simulink model "dve_nadrze_linearized"  (R2016a)
settings: Solver=VariableStepAuto  SolverMode=SingleTasking  StartTime=0.0  StopTime=t  RelTol=1e-3
undefined symbols (not defined in the file): A, B, C, D, dQ, H1r, H2r, stepTime, U
settings Model: Creator=Filip Jašek  LastModifiedBy=Filip Jašek
settings DataIOCC: ReturnWorkspaceOutputs=on
settings DebuggingCC: SFUnexpectedBacktrackingDiag=error  SFNoUnconditionalDefaultTransitionDiag=error
settings SFSimCC: SimUseLocalCustomCode=on
settings RTWCC: RTWUseLocalCustomCode=on
settings GRTTargetCC: TargetLangStandard=C99 (ISO)
settings ConfigComp: CovMetricSettings=dwe  CovHtmlReporting=off  CovSaveCumulativeToWorkspaceVar=off  CovSaveSingleToWorkspaceVar=off  CovExternalEMLEnable=on

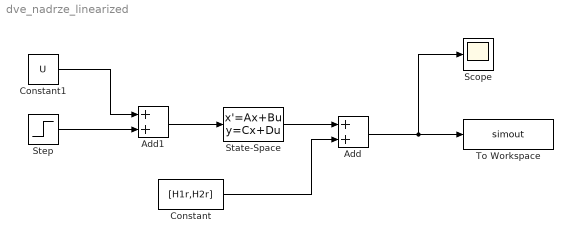
== system dve_nadrze_linearized ==
  Add : Sum
  Add1 : Sum
  Constant : Constant  Value=[H1r,H2r]
  Constant1 : Constant  Value=U
  Scope : Scope
  State-Space : StateSpace  A=A  B=B  C=C  D=D  X0=0
  Step : Step  Time=stepTime  After=dQ  SampleTime=0
  To Workspace : ToWorkspace  VariableName=simout  SaveFormat=Timeseries  SampleTime=-1
  wires:
  State-Space/1 -> Add/1
  Constant/1 -> Add/2
  Add/1 -> Scope/1, To Workspace/1
  Constant1/1 -> Add1/1
  Step/1 -> Add1/2
  Add1/1 -> State-Space/1
